simulink model "simulation_control_observer_state_feedback_WP3"  (R2023b)
settings: Solver=VariableStepAuto  StartTime=0.0  StopTime=100  RelTol=1e-3
values from neighbouring files (symbols this model uses):
  A = [0 1; 9.81 -0.1]    [WP3.m]
  B = [0; 1]    [WP3.m]
  C = [1 0]    [WP3.m]
  K = [92.0469   14.4179]    [WP3.m]
  L = [l1; l2]    [WP3.m]
  r = simOut.get('r')    [plotSimulationResults.m]
undefined symbols (not defined in the file or in its folder): kr
settings Model: Creator=giova  LastModifiedBy=michele

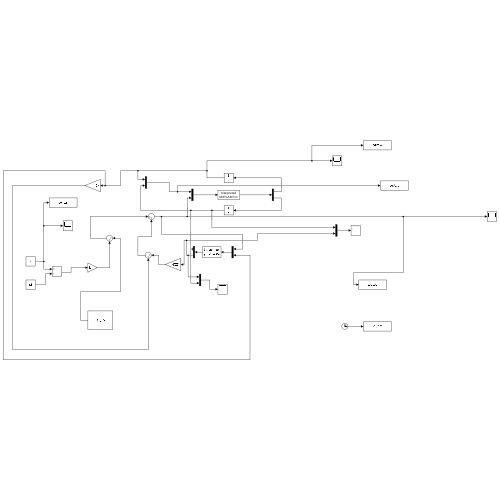
[thumbnail: Simulink's stored preview of the top-level diagram]
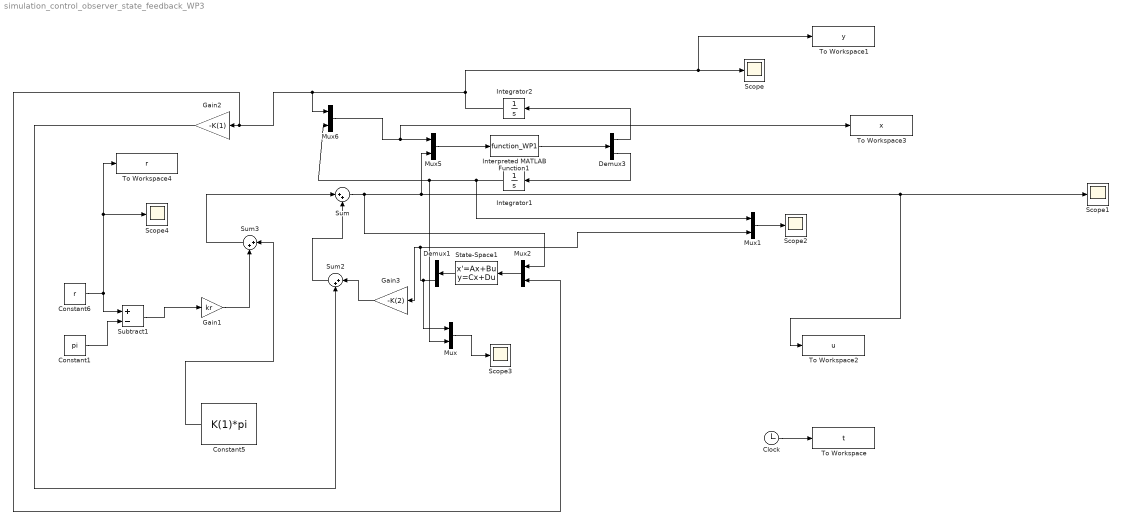
== system simulation_control_observer_state_feedback_WP3 ==
  Clock : Clock
  Constant1 : Constant  Value=pi
  Constant5 : Constant  Value=K(1)*pi
  Constant6 : Constant  Value=r
  Demux1 : Demux  Outputs=2
  Demux3 : Demux  Outputs=2
  Gain1 : Gain  Gain=kr
  Gain2 : Gain  Gain=-K(1)
  Gain3 : Gain  Gain=-K(2)
  Integrator1 : Integrator
  Integrator2 : Integrator
  Interpreted MATLAB Function1 : MATLABFcn  MATLABFcn=function_WP1  OutputDimensions=2
  Mux{,1..2,5..6} (5 alike) : Mux  Inputs=2
  Scope{,1..4} (5 alike) : Scope
  State-Space1 : StateSpace  A=A-L*C  B=[B L]  C=eye(2)  D=[0 0; 0 0]  InitialCondition=[0 0]
  Subtract1 : Sum  Inputs=+-
  Sum : Sum  Inputs=|++
  Sum2 : Sum  Inputs=|++
  Sum3 : Sum  Inputs=|++
  To Workspace : ToWorkspace  VariableName=t  SampleTime=-1
  To Workspace1 : ToWorkspace  VariableName=y  SampleTime=-1
  To Workspace2 : ToWorkspace  VariableName=u  SampleTime=-1
  To Workspace3 : ToWorkspace  VariableName=x  SampleTime=-1
  To Workspace4 : ToWorkspace  VariableName=r  SampleTime=-1
  wires:
  Demux1/2 -> Mux/1, Mux1/2, Gain3/1
  State-Space1/1 -> Demux1/1
  Gain3/1 -> Sum2/1
  Gain2/1 -> Sum2/2
  Sum2/1 -> Sum/2
  Mux2/1 -> State-Space1/1
  Sum/1 -> To Workspace2/1, Scope1/1, Mux5/2, Mux2/1
  Mux5/1 -> Interpreted MATLAB Function1/1
  Interpreted MATLAB Function1/1 -> Demux3/1
  Demux3/1 -> Integrator2/1
  Integrator2/1 -> Mux2/2, Gain2/1, Mux6/1, To Workspace1/1, Scope/1
  Mux6/1 -> To Workspace3/1, Mux5/1
  Clock/1 -> To Workspace/1
  Demux3/2 -> Integrator1/1
  Integrator1/1 -> Mux1/1, Mux/2, Mux6/2
  Mux1/1 -> Scope2/1
  Constant1/1 -> Subtract1/2
  Gain1/1 -> Sum3/2
  Constant5/1 -> Sum3/1
  Constant6/1 -> Subtract1/1, To Workspace4/1, Scope4/1
  Subtract1/1 -> Gain1/1
  Sum3/1 -> Sum/1
  Mux/1 -> Scope3/1
